simulink model "TwoMasssystemRigid_v1"  (Simulink 7.0)
settings: Solver=ode4  StartTime=0.0  StopTime=tstop  FixedStep=h_v1  RelTol=1e-3
values from neighbouring files (symbols this model uses):
  f = 10    [main.m]
  Fmax = 100    [main.m]
  m1 = 0.1    [main.m]
  m2 = 0.2    [main.m]
  x1_0 = x3_0    (= 0)    [main.m]
  x2_0 = x4_0    (= 0)    [main.m]
  x3_0 = 0    [main.m]
  x4_0 = 0    [main.m]
settings Model: Creator=adminus  LastModifiedBy=adminus

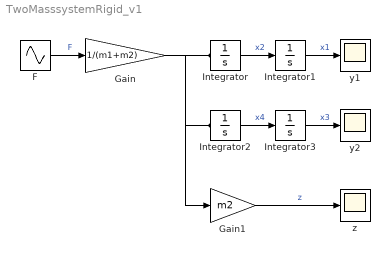
== system TwoMasssystemRigid_v1 ==
  F : Sin  Amplitude=Fmax  Frequency=2*pi*f  SampleTime=0
  Gain : Gain  Gain=1/(m1+m2)  ParameterDataType=sfix(16)  ParameterScaling=2^0  OutDataType=sfix(16)  OutScaling=2^0
  Gain1 : Gain  Gain=m2  ParameterDataType=sfix(16)  ParameterScaling=2^0  OutDataType=sfix(16)  OutScaling=2^0
  Integrator : Integrator  InitialCondition=x2_0
  Integrator1 : Integrator  InitialCondition=x1_0
  Integrator2 : Integrator  InitialCondition=x4_0
  Integrator3 : Integrator  InitialCondition=x3_0
  y1 : Scope
      settings: TimeRange=10  SaveName=ScopeData_v1_y1
  y2 : Scope
  z : Scope
      settings: SaveName=ScopeData2
  wires:
  F/1 -> Gain/1  "F"
  Gain/1 -> Integrator/1, Integrator2/1, Gain1/1
  Integrator/1 -> Integrator1/1  "x2"
  Integrator1/1 -> y1/1  "x1"
  Integrator2/1 -> Integrator3/1  "x4"
  Integrator3/1 -> y2/1  "x3"
  Gain1/1 -> z/1  "z"
